simulink model "pokus_1"  (Simulink 7.3)
settings: Solver=ode1  SolverMode=SingleTasking  StartTime=0.0  StopTime=10.0  FixedStep=0.001  RelTol=1e-3
PostLoadFcn:
  | run('parametri.m');
values from neighbouring files (symbols this model uses):
  Beq = 0.004    [all_the_data.mat]    (also in parametri.m)
  Eff_G = 0.9    [all_the_data.mat]    (also in parametri.m)
  Eff_M = 0.69    [all_the_data.mat]    (also in parametri.m)
  Jeq = 0.002    [all_the_data.mat]    (also in parametri.m)
  Ke = 0.0076776    [all_the_data.mat]    (also in parametri.m)
  Kg = 70    [all_the_data.mat]    (also in parametri.m)
  Km = 0.007683    [all_the_data.mat]    (also in parametri.m)
  Kp = 29.3398872208    [all_the_data.mat]    (also in parametri.m)
  Kv = 0.364280264132    [all_the_data.mat]    (also in parametri.m)
  Ra = 2.6    [all_the_data.mat]    (also in parametri.m)
undefined symbols (not defined in the file or in its folder): MultiQ, PCI, Quanser
libraries: rtwinlib x2
settings Model: Creator=Niko  LastModifiedBy=Mehatronicki Sustavi  SimulationMode=external  ExtModeTrigDuration=10001
settings DebuggingCC: StrictBusMsg=ErrorLevel1
settings HardwareCC: ProdIntDivRoundTo=Zero  ProdEndianess=LittleEndian  ProdHWDeviceType=Generic->32-bit x86 compatible
settings RTWCC: SystemTargetFile=rtwin.tlc  TemplateMakefile=rtwin.tmf  Description=Real-Time Windows Target  ProcessScript=rtwin_make_rtw_hook  RTWCompilerOptimization=On
settings CodeAppCC: MaxIdLength=95
settings RTWinTargetCC: TargetFunctionLibrary=ANSI_C  PortableWordSizes=off

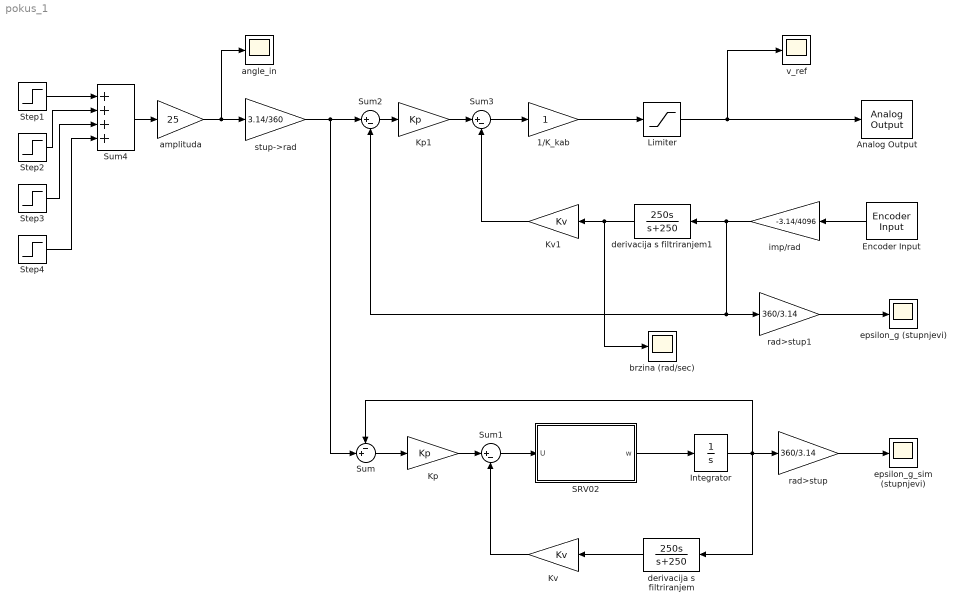
== system pokus_1 ==
  " derivacija s filtriranjem" : TransferFcn  Numerator=[250 0]  Denominator=[1 250]
  " derivacija s filtriranjem1" : TransferFcn  Numerator=[250 0]  Denominator=[1 250]
  1/K_kab : Gain
  Analog Output : rtwinlib/Analog Output  SampleTime=0.001  DrvName=Quanser/MultiQ-PCI  DrvAddress=4294967295  DrvOptions=zeros(1,0)  Channels=1  RangeMode=1  VoltRange=1  InitialValue=0  FinalValue=0
      settings: AttributesFormatString=Quanser\nMultiQ-PCI [auto]
  Encoder Input : rtwinlib/Encoder Input  SampleTime=-1  DrvName=Quanser/MultiQ-PCI  DrvAddress=4294967295  DrvOptions=zeros(1,0)  Channels=1  QuadMode=3  IndexPulse=2  InputFilter=Inf  DataType=1
      settings: AttributesFormatString=Quanser\nMultiQ-PCI [auto]
  Integrator : Integrator
  Kp : Gain  Gain=Kp
  Kp1 : Gain  Gain=Kp
  Kv : Gain  Gain=Kv
  Kv1 : Gain  Gain=Kv
  Limiter : Saturate  UpperLimit=6  LowerLimit=-6
  SRV02 : Subsystem
  Step1 : Step
  Step2 : Step  Time=2  After=-1
  Step3 : Step  Time=3  After=-1
  Step4 : Step  Time=4
  Sum : Sum  Inputs=-+|
  Sum1 : Sum  Inputs=|+-
  Sum2 : Sum  Inputs=|+-
  Sum3 : Sum  Inputs=|+-
  Sum4 : Sum  Inputs=++++
  amplituda : Gain  Gain=25
  angle_in : Scope
      settings: TimeRange=5  YMin=-1  YMax=1  SaveName=angle_in  DataFormat=Array  SampleInput=on
  brzina (rad/sec) : Scope
      settings: TimeRange=5  YMin=0  YMax=30  SaveName=brzina  DataFormat=Array  SampleInput=on
  epsilon_g (stupnjevi) : Scope
      settings: TimeRange=5  YMin=0  YMax=30  SaveName=epsi_g  DataFormat=Array  SampleInput=on
  epsilon_g_sim (stupnjevi) : Scope
      settings: TimeRange=5  YMin=0  YMax=30  SaveName=epsi_g_sim  DataFormat=Array  SampleInput=on
  imp/rad : Gain  Gain=-3.14/4096
  rad>stup : Gain  Gain=360/3.14
  rad>stup1 : Gain  Gain=360/3.14
  stup->rad : Gain  Gain=3.14/360
  v_ref : Scope
      settings: TimeRange=5  YMin=0  YMax=30  SaveName=v_ref  DataFormat=Array  SampleInput=on
  wires:
  Integrator/1 -> rad>stup/1, Sum/1, " derivacija s filtriranjem"/1
  Kp/1 -> Sum1/1
  Sum/1 -> Kp/1
  " derivacija s filtriranjem"/1 -> Kv/1
  Kv/1 -> Sum1/2
  Sum1/1 -> SRV02/1(U)
  SRV02/1(w) -> Integrator/1
  stup->rad/1 -> Sum/2, Sum2/1
  rad>stup/1 -> epsilon_g_sim (stupnjevi)/1
  Kp1/1 -> Sum3/1
  Sum2/1 -> Kp1/1
  " derivacija s filtriranjem1"/1 -> brzina (rad/sec)/1, Kv1/1
  Kv1/1 -> Sum3/2
  Sum3/1 -> 1/K_kab/1
  Limiter/1 -> v_ref/1, Analog Output/1
  1/K_kab/1 -> Limiter/1
  imp/rad/1 -> rad>stup1/1, Sum2/2, " derivacija s filtriranjem1"/1
  rad>stup1/1 -> epsilon_g (stupnjevi)/1
  Sum4/1 -> amplituda/1
  Step4/1 -> Sum4/4
  Step3/1 -> Sum4/3
  Step2/1 -> Sum4/2
  Step1/1 -> Sum4/1
  amplituda/1 -> angle_in/1, stup->rad/1
  Encoder Input/1 -> imp/rad/1

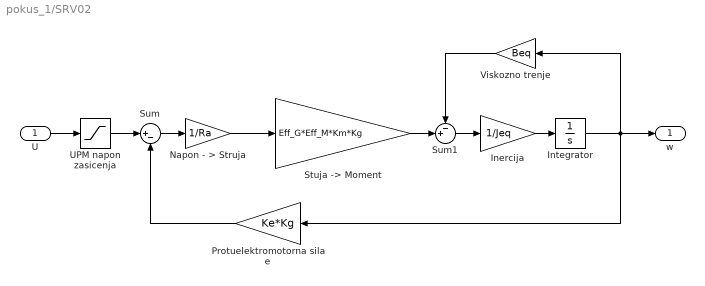
== system pokus_1/SRV02 ==
  U : Inport
  Inercija : Gain  Gain=1/Jeq
  Integrator : Integrator
  Napon - > Struja : Gain  Gain=1/Ra
  Protuelektromotorna sila e : Gain  Gain=Ke*Kg
  "Stuja -> Moment" : Gain  Gain=Eff_G*Eff_M*Km*Kg
  Sum : Sum  Inputs=|+-
  Sum1 : Sum  Inputs=-+|
  UPM napon zasicenja : Saturate  UpperLimit=6  LowerLimit=-6
  Viskozno trenje : Gain  Gain=Beq
  w : Outport
  wires:
  Sum1/1 -> Inercija/1
  "Stuja -> Moment"/1 -> Sum1/2
  Inercija/1 -> Integrator/1
  UPM napon zasicenja/1 -> Sum/1
  Napon - > Struja/1 -> "Stuja -> Moment"/1
  U/1 -> UPM napon zasicenja/1
  Sum/1 -> Napon - > Struja/1
  Viskozno trenje/1 -> Sum1/1
  Protuelektromotorna sila e/1 -> Sum/2
  Integrator/1 -> w/1, Protuelektromotorna sila e/1, Viskozno trenje/1
